simulink model "solo"  (R2020a)
settings: Solver=VariableStepAuto  StartTime=0.0  StopTime=100  RelTol=1e-3
settings Model: Creator=josem  LastModifiedBy=josem

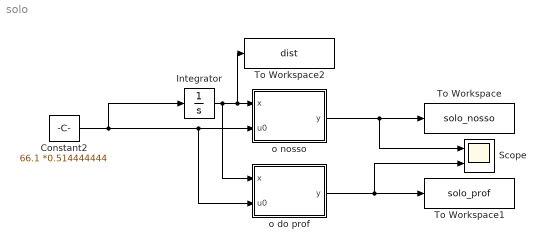
== system solo ==
  Constant2 : Constant  Value=66.1 *0.514444444
  Integrator : Integrator
  Scope : Scope  NumInputPorts=2
  To Workspace : ToWorkspace  VariableName=solo_nosso  SampleTime=-1
  To Workspace1 : ToWorkspace  VariableName=solo_prof  SampleTime=-1
  To Workspace2 : ToWorkspace  VariableName=dist  SampleTime=-1
  o do prof : MATLAB Function  TreatAsAtomicUnit=on
  o nosso : MATLAB Function  TreatAsAtomicUnit=on
  wires:
  Constant2/1 -> Integrator/1, o do prof/2(u0), o nosso/2(u0)
  Integrator/1 -> o do prof/1(x), To Workspace2/1, o nosso/1(x)
  o nosso/1(y) -> To Workspace/1, Scope/1
  o do prof/1(y) -> To Workspace1/1, Scope/2

== matlab function solo/o nosso ==
  data: x input; y output; u0 input
function y = fcn(x, u0)

% if (u<20*u0)
%    y=(-5/20)*u+5*u0;
% elseif (20*u0<=u) && (u<40*u0)
%    y=0;
% elseif (40*u0<=u) && (u<60*u0)
%    %y=2.5*u0*sin((3.14159265359/(20*u0))*u) +2.5*u0;
%    y=5*u0*sin(((u/(20*u0))-2)*pi/2);
% 
% else
%     
%    y=5*u0;

if (x<40*u0)
   y=(-5/40)*x+5*u0+100;
   
elseif (40*u0<=x) && (x<60*u0)
   y=100;
   
elseif (60*u0<=x) && (x<100*u0)
   %y=2.5*u0*sin((3.14159265359/(20*u0))*u) +2.5*u0;
   %y=5*u0*sin(((u/(20*u0))-2)*pi/2);
   amplitude = 50; %(m)
   periodo = 40*2; %meio periodo sao 40s
   offset = +50;
   y=offset+amplitude*sin(2*pi/(periodo*u0)*(x-60*u0)+pi/2);

else
    
   y=0;
end

== matlab function solo/o do prof ==
  data: x input; y output; u0 input
function y = fcn(x, u0)

% if (u<20*u0)
%    y=(-5/20)*u+5*u0;
% elseif (20*u0<=u) && (u<40*u0)
%    y=0;
% elseif (40*u0<=u) && (u<60*u0)
%    %y=2.5*u0*sin((3.14159265359/(20*u0))*u) +2.5*u0;
%    y=5*u0*sin(((u/(20*u0))-2)*pi/2);
% 
% else
%     
%    y=5*u0;
if (x<20*u0)
   y=(-5/20)*x+5*u0;
   
elseif (20*u0<=x) && (x<40*u0)
   y=0;
   
elseif (40*u0<=x) && (x<60*u0)
   %y=2.5*u0*sin((3.14159265359/(20*u0))*u) +2.5*u0;
   %y=5*u0*sin(((u/(20*u0))-2)*pi/2);
   amplitude = 5*u0/2; %(m)
   periodo = 20*2; %meio periodo sao 20s
   offset = +amplitude;
   y=offset+amplitude*sin(2*pi/(periodo*u0)*(x-40*u0)-pi/2);

elseif (60*u0<=x) && (x<80*u0)
   y=5*u0;
   
else
    
   y=5*u0;
end
